simulink model "untitled"  (R2016a)
settings: Solver=VariableStepAuto  SolverMode=SingleTasking  StartTime=0.0  StopTime=10.0  RelTol=1e-3
values from neighbouring files (symbols this model uses):
  A = [0 1 0 0 0 0 0 0 ... (first row only)    [dynamics_simple.m]
  AA = A-B*K    [dynamics_simple.m]
  B = [0 0 ... (first row only)    [dynamics_simple.m]
  C = [1 0 0 0 0 0 0 0 ... (first row only)    [dynamics_simple.m]
  D = [0 0;0 0;0 0;0 0;0 0;0 0;0 0;0 0]    [dynamics_simple.m]
  K = place(A,B,P)    [dynamics_simple.m]
settings Model: Creator=apple  LastModifiedBy=16171
settings DebuggingCC: SFUnexpectedBacktrackingDiag=error  SFNoUnconditionalDefaultTransitionDiag=error
settings GRTTargetCC: TargetLangStandard=C99 (ISO)  GeneratePreprocessorConditionals=Use local settings
settings ConfigComp: CovMetricSettings=dwe  CovHtmlReporting=off  CovSaveCumulativeToWorkspaceVar=off  CovSaveSingleToWorkspaceVar=off  CovExternalEMLEnable=on

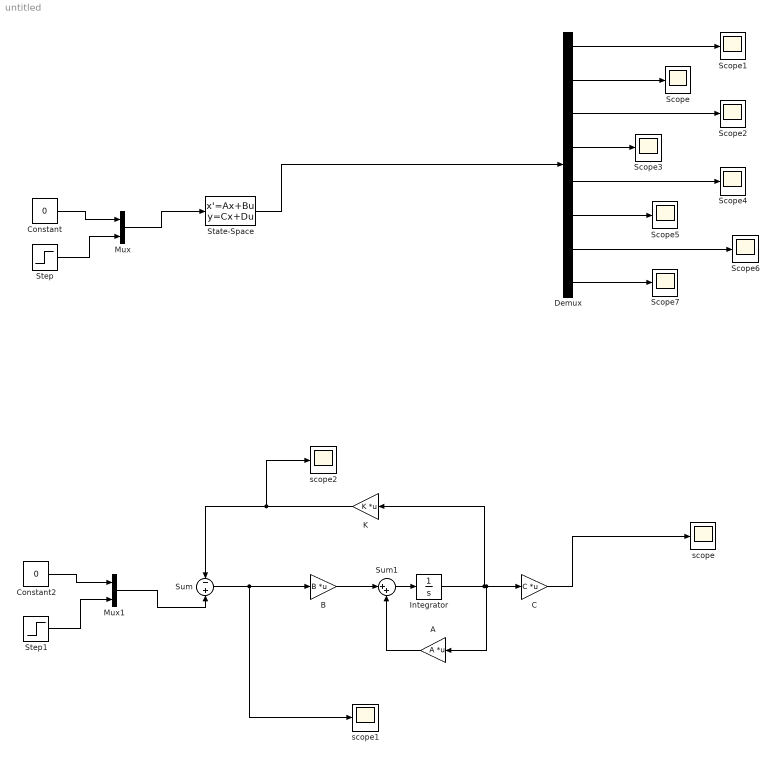
== system untitled ==
  A : Gain  Gain=A  Multiplication=Matrix(K*u)
  B : Gain  Gain=B  Multiplication=Matrix(K*u)
  C : Gain  Gain=C  Multiplication=Matrix(K*u)
  Constant : Constant  Value=0
  Constant2 : Constant  Value=0
  Demux : Demux  Outputs=8
  Integrator : Integrator
  K : Gain  Gain=K  Multiplication=Matrix(K*u)
  Mux : Mux  Inputs=2
  Mux1 : Mux  Inputs=2
  Scope{,1..7} (8 alike) : Scope
  State-Space : StateSpace  A=AA  B=B  C=C  D=D  X0=[0 0 0 0 0 0 0 0]
  Step : Step  SampleTime=0
  Step1 : Step  Time=0  SampleTime=0
  Sum : Sum  Inputs=-+
  Sum1 : Sum  Inputs=|++
  scope : Scope
  scope1 : Scope
  scope2 : Scope
  wires:
  State-Space/1 -> Demux/1
  Step/1 -> Mux/2
  Constant/1 -> Mux/1
  Mux/1 -> State-Space/1
  Demux/2 -> Scope/1
  Demux/8 -> Scope7/1
  Demux/1 -> Scope1/1
  Demux/3 -> Scope2/1
  Demux/4 -> Scope3/1
  Demux/5 -> Scope4/1
  Demux/6 -> Scope5/1
  Demux/7 -> Scope6/1
  Sum1/1 -> Integrator/1
  B/1 -> Sum1/1
  A/1 -> Sum1/2
  C/1 -> scope/1
  Integrator/1 -> K/1, A/1, C/1
  Step1/1 -> Mux1/2
  Constant2/1 -> Mux1/1
  Mux1/1 -> Sum/2
  K/1 -> scope2/1, Sum/1
  Sum/1 -> scope1/1, B/1
